simulink model "workingNonlinearFunc"  (R2022b)
settings: Solver=VariableStepAuto  StartTime=0.0  StopTime=10  RelTol=1e-3
settings Model: Creator=darcyschofield  LastModifiedBy=darcyschofield

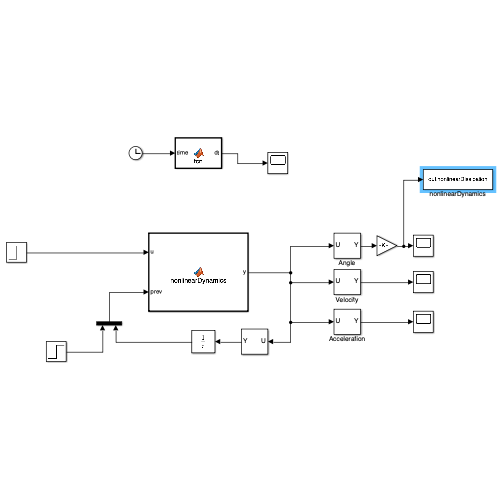
[thumbnail: Simulink's stored preview of the top-level diagram]
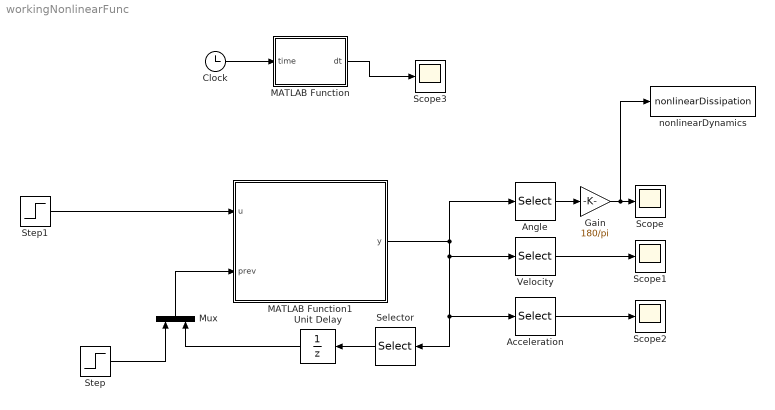
== system workingNonlinearFunc ==
  Acceleration : Selector  InputPortWidth=9  IndexOptions=Index vector (dialog)  Indices=[7 8 9]  OutputSizes=1
  Angle : Selector  InputPortWidth=9  IndexOptions=Index vector (dialog)  Indices=[1 2 3]  OutputSizes=1
  Clock : Clock
  Gain : Gain  Gain=180/pi
  MATLAB Function : MATLAB Function  TreatAsAtomicUnit=on
  MATLAB Function1 : MATLAB Function  TreatAsAtomicUnit=on
  Mux : Mux  Inputs=2
  Scope{,1..3} (4 alike) : Scope
  Selector : Selector  InputPortWidth=9  IndexOptions=Index vector (dialog)  Indices=[7 8 9]  OutputSizes=1
  Step : Step  Time=0  After=[1; 1; 1; 1; 1; 1]  SampleTime=0
  Step1 : Step  Time=0  After=[0; 0; 0]  SampleTime=0
  Unit Delay : UnitDelay  InitialCondition=[0; 0; 0]  SampleTime=-1  HasFrameUpgradeWarning=on
  Velocity : Selector  InputPortWidth=9  IndexOptions=Index vector (dialog)  Indices=[4 5 6]  OutputSizes=1
  nonlinearDynamics : ToWorkspace  VariableName=nonlinearDissipation  SaveFormat=Timeseries  SampleTime=-1
  wires:
  Clock/1 -> MATLAB Function/1(time)
  Step1/1 -> MATLAB Function1/1(u)
  Acceleration/1 -> Scope2/1
  Velocity/1 -> Scope1/1
  MATLAB Function/1(dt) -> Scope3/1
  Angle/1 -> Gain/1
  Gain/1 -> nonlinearDynamics/1, Scope/1
  MATLAB Function1/1(y) -> Angle/1, Velocity/1, Selector/1, Acceleration/1
  Unit Delay/1 -> Mux/2
  Mux/1 -> MATLAB Function1/2(prev)
  Step/1 -> Mux/1
  Selector/1 -> Unit Delay/1

== matlab function workingNonlinearFunc/MATLAB Function1 ==
  data: u input; y output; prev input
function y = nonlinearDynamics(u, prev)
% Vectorized discrete dynamics for a 3-link planar robot leg

% x_prev: 6x1 state vector = [q1; q2; q3; dq1; dq2; dq3]
% u_prev: 3x1 torque vector = [tau1; tau2; tau3]
% ddq_prev: 3x1 vector of previous accelerations
% dt: scalar time step

% Unpack inputs
q = prev(1:3);
dq = prev(4:6);
ddq_prev = prev(7:9);

tau = u;

q1 = q(1); q2 = q(2); q3 = q(3);
dq1 = dq(1); dq2 = dq(2); dq3 = dq(3);
tau1 = tau(1); tau2 = tau(2); tau3 = tau(3);
ddq1_prev = ddq_prev(1); ddq2_prev = ddq_prev(2); ddq3_prev = ddq_prev(3);

% Damping coeffs
b1 = 1;
b2 = 1;
b3 = 1;


ddq1 = (-5000000.0*b1*dq1 - 325845.0*ddq2_prev*cos(q2 + q3) - 2983860.0*ddq2_prev*cos(q2) - 637208.0*ddq2_prev*cos(q3) - 2092085.0*ddq2_prev...
        - 325845.0*ddq3_prev*cos(q2 + q3) - 318604.0*ddq3_prev*cos(q3) - 94133.0*ddq3_prev + 651690.0*dq1*dq2*sin(q2 + q3)...
        + 5967720.0*dq1*dq2*sin(q2) + 651690.0*dq1*dq3*sin(q2 + q3) + 637208.0*dq1*dq3*sin(q3) + 325845.0*dq2^2*sin(q2 + q3)...
        + 2983860.0*dq2^2*sin(q2) + 651690.0*dq2*dq3*sin(q2 + q3) + 637208.0*dq2*dq3*sin(q3) + 325845.0*dq3^2*sin(q2 + q3)...
        + 318604.0*dq3^2*sin(q3) + 5000000.0*tau1 + 65048148.0*cos(q1 + q2) + 7103421.0*cos(q1 + q2 + q3)...
        + 201168765.0*cos(q1))/(651690.0*cos(q2 + q3) + 5967720.0*cos(q2) + 637208.0*cos(q3) + 9193760.0);

ddq2 = (-5000000.0*b2*dq2 - 325845.0*ddq1_prev*cos(q2 + q3) - 2983860.0*ddq1_prev*cos(q2) - 637208.0*ddq1_prev*cos(q3) - 2092085.0*ddq1_prev...
        - 318604.0*ddq3_prev*cos(q3) - 94133.0*ddq3_prev - 325845.0*dq1^2*sin(q2 + q3) - 2983860.0*dq1^2*sin(q2)... 
        + 637208.0*dq1*dq3*sin(q3) + 637208.0*dq2*dq3*sin(q3) + 318604.0*dq3^2*sin(q3) + 5000000.0*tau2...
        + 65048148.0*cos(q1 + q2) + 7103421.0*cos(q1 + q2 + q3))/(637208.0*cos(q3) + 2092085.0);

ddq3 = -53.1163353977882*b3*dq3 - 3.46153846153846*ddq1_prev*cos(q2 + q3) - 3.38461538461538*ddq1_prev*cos(q3) - ddq1_prev... 
        - 3.38461538461538*ddq2_prev*cos(q3) - ddq2_prev - 3.46153846153846*dq1^2*sin(q2 + q3) - 3.38461538461538*dq1^2*sin(q3)... 
        - 6.76923076923077*dq1*dq2*sin(q3) - 3.38461538461538*dq2^2*sin(q3) + 53.1163353977882*tau3 + 75.4615384615385*cos(q1 + q2 + q3);

ddq = [ddq1; ddq2; ddq3];

% --- Discrete integration ---
dt = 0.01;
dq_next = dq + dt * ddq;
q_next  = q  + dt * dq_next;

y = [q_next; dq_next; ddq];

end

== matlab function workingNonlinearFunc/MATLAB Function ==
  data: time input; dt output
function dt = fcn(time)
    persistent prev_time

    if isempty(prev_time)
        prev_time = time;  % initialize
        dt = 0;
    else
        dt = time - prev_time;
        prev_time = time;
    end
end
